simulink model "Older_model_ contains_ACC"  (R2023b)
settings: Solver=VariableStepAuto  StartTime=0.0  StopTime=30  MaxStep=1e-2  RelTol=1e-3  AbsTol=1e-3
values from neighbouring files (symbols this model uses):
  b = 1.6    [a2024_v2x_matlab_6veh.m]
  m = 2000    [a2024_v2x_matlab_6veh.m]
  mEgo = 1500    [a2024_v2x_matlab_6veh.m]
  sampleTime = 0.1    [a2024_v2x_matlab_6veh.m]    (also in v2x_matlab.m; v2x_matlabV2.m; v2x_matlab_6veh.m; v2x_matlab_R.m)
  t_gap = 1.4    [a2024_v2x_matlab_6veh.m]
  waypoints = [egoWP(:,2) egoWP(:,1), zeroforwp]    [a2024_v2x_matlab_6veh.m]    (also in misc.m = data.data.ActorSpecifications(1,1).Waypoints(:,[1,2]); v2x_matlab.m = data.data.ActorSpecifications(1,1).Waypoints(:,[1,2]); v2x_matlabV2.m = [5 -1.6 0; v2x_matlab_R.m = [5 -1.6 0)
  ZeroActors = struct(     'ActorID',0,     'Position', [1000 1000 1000],      'Velocity', [0 0 0],      'Roll', 0,      'Pitch', 0,      'Yaw', 0,      'AngularVelocity', [0 0 0])    [v2x_matlabV2.m]    (also in v2x_matlab_R.m)
undefined symbols (not defined in the file or in its folder): doppler, driving, n, PredictionHorizon, Ts
libraries: simulink x13, simulink_extras x12, commofdm x10, commdigbbndam3 x10, commchan3 x3, drivingscenarioandsensors x3, mpcadaslib x2, commsink2 x2, vehdynlibdriver x1, dspmathops x1, autolibshared x1
(part 2 of 3)

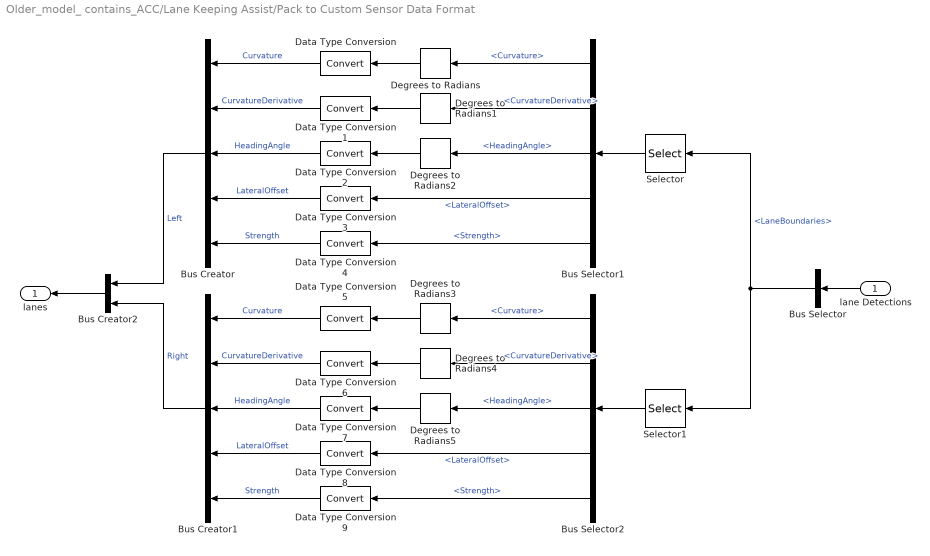
== system Older_model_ contains_ACC/Lane Keeping Assist/Pack to Custom Sensor Data Format ==
  lane Detections : Inport
  Bus Creator : BusCreator  Inputs=5
  Bus Creator1 : BusCreator  Inputs=5
  Bus Creator2 : BusCreator  Inputs=2
  Bus Selector : BusSelector  OutputSignals=LaneBoundaries
  Bus Selector1 : BusSelector  OutputSignals=Curvature,CurvatureDerivative,HeadingAngle,LateralOffset,Strength
  Bus Selector2 : BusSelector  OutputSignals=Curvature,CurvatureDerivative,HeadingAngle,LateralOffset,Strength
  Data Type Conversion{,1..9} (10 alike) : DataTypeConversion  SaturateOnIntegerOverflow=off  RndMeth=Floor
  Degrees to Radians{,1..5} (6 alike) : simulink_extras/Transformations/Degrees to Radians
  Selector : Selector  IndexMode=Zero-based  InputPortWidth=30  IndexOptions=Index vector (dialog)  Indices=1  OutputSizes=1
  Selector1 : Selector  InputPortWidth=30  IndexOptions=Index vector (dialog)  Indices=2  OutputSizes=1
  lanes : Outport  VectorParamsAs1DForOutWhenUnconnected=off
  wires:
  lane Detections/1 -> Bus Selector/1
  Bus Selector/1 -> Selector/1, Selector1/1  "<LaneBoundaries>"
  Selector/1 -> Bus Selector1/1
  Bus Selector1/2 -> Degrees to Radians1/1  "<CurvatureDerivative>"
  Bus Selector1/1 -> Degrees to Radians/1  "<Curvature>"
  Bus Selector1/3 -> Degrees to Radians2/1  "<HeadingAngle>"
  Degrees to Radians/1 -> Data Type Conversion/1
  Degrees to Radians1/1 -> Data Type Conversion1/1
  Degrees to Radians2/1 -> Data Type Conversion2/1
  Bus Selector1/4 -> Data Type Conversion3/1  "<LateralOffset>"
  Bus Selector1/5 -> Data Type Conversion4/1  "<Strength>"
  Data Type Conversion/1 -> Bus Creator/1  "Curvature"
  Data Type Conversion1/1 -> Bus Creator/2  "CurvatureDerivative"
  Data Type Conversion2/1 -> Bus Creator/3  "HeadingAngle"
  Data Type Conversion3/1 -> Bus Creator/4  "LateralOffset"
  Data Type Conversion4/1 -> Bus Creator/5  "Strength"
  Data Type Conversion9/1 -> Bus Creator1/5  "Strength"
  Data Type Conversion6/1 -> Bus Creator1/2  "CurvatureDerivative"
  Data Type Conversion7/1 -> Bus Creator1/3  "HeadingAngle"
  Data Type Conversion8/1 -> Bus Creator1/4  "LateralOffset"
  Data Type Conversion5/1 -> Bus Creator1/1  "Curvature"
  Bus Selector2/1 -> Degrees to Radians3/1  "<Curvature>"
  Selector1/1 -> Bus Selector2/1
  Bus Selector2/4 -> Data Type Conversion8/1  "<LateralOffset>"
  Bus Selector2/5 -> Data Type Conversion9/1  "<Strength>"
  Bus Selector2/2 -> Degrees to Radians4/1  "<CurvatureDerivative>"
  Degrees to Radians5/1 -> Data Type Conversion7/1
  Degrees to Radians3/1 -> Data Type Conversion5/1
  Degrees to Radians4/1 -> Data Type Conversion6/1
  Bus Selector2/3 -> Degrees to Radians5/1  "<HeadingAngle>"
  Bus Creator2/1 -> lanes/1
  Bus Creator/1 -> Bus Creator2/1  "Left"
  Bus Creator1/1 -> Bus Creator2/2  "Right"

== system Older_model_ contains_ACC/Lane Keeping Assist/Subsystem ==
  Lane Assist Offset : Inport
  Lane Sensor data : Inport  Port=2
  Bus Selector3 : BusSelector  OutputSignals=Left.LateralOffset,Right.LateralOffset
  Gain3 : Gain  Gain=-1
  Logical Operator : Logic  Operator=OR  AllPortsSameDT=off  OutDataTypeStr=boolean
  Relational Operator : RelationalOperator  Operator=<=  OutDataTypeStr=boolean  RndMeth=Simplest  InputSameDT=off
  Relational Operator1 : RelationalOperator  OutDataTypeStr=boolean  RndMeth=Simplest  InputSameDT=off
  Departure Detected : Outport
  wires:
  Relational Operator1/1 -> Logical Operator/2
  Bus Selector3/2 -> Relational Operator1/1  "<LateralOffset>"
  Bus Selector3/1 -> Relational Operator/1  "<LateralOffset>"
  Relational Operator/1 -> Logical Operator/1
  Logical Operator/1 -> Departure Detected/1
  Gain3/1 -> Relational Operator1/2
  Lane Assist Offset/1 -> Gain3/1, Relational Operator/2
  Lane Sensor data/1 -> Bus Selector3/1

== system Older_model_ contains_ACC/Lane Keeping Assist/Subsystem2 ==
  Enable : Inport
  Set : Inport  Port=2
  Assisted Steer : Inport  Port=3
  Driver Steer : Inport  Port=4
  AND : Logic  IconShape=distinctive  AllPortsSameDT=off  OutDataTypeStr=boolean
  Latch Assist : Subsystem
  Subsystem1 : Subsystem
  Switch : Switch  Criteria=u2 > Threshold  SaturateOnIntegerOverflow=off  InputSameDT=off
  Status : Outport
  SteeringAngle in rad : Outport  Port=2
  wires:
  Enable/1 -> AND/1
  AND/1 -> Status/1, Switch/2
  Latch Assist/1(Assist) -> AND/2
  Subsystem1/1(Similar) -> Latch Assist/2(Reset)
  Driver Steer/1 -> Switch/3, Subsystem1/2(Driver Steer)
  Assisted Steer/1 -> Switch/1, Subsystem1/1(Assisted Steer)
  Switch/1 -> SteeringAngle in rad/1
  Set/1 -> Latch Assist/1(Set)

== system Older_model_ contains_ACC/Subsystem3/If Action Subsystem ==
  In1 : Inport
  Action Port : ActionPort  ActionPortLabel=case [ 1 ]:
  Out1 : Outport
  wires:
  In1/1 -> Out1/1

== system Older_model_ contains_ACC/Subsystem3/If Action Subsystem1 ==
  In1 : Inport
  Action Port : ActionPort  ActionPortLabel=case [ 2 ]:
  Out1 : Outport
  wires:
  In1/1 -> Out1/1

== system Older_model_ contains_ACC/Subsystem3/If Action Subsystem2 ==
  Actors : Inport
  Action Port : ActionPort  ActionPortLabel=case [ 3 ]:
  Out1 : Outport
  wires:
  Actors/1 -> Out1/1

== system Older_model_ contains_ACC/Subsystem3/If Action Subsystem3 ==
  Actors : Inport
  Action Port : ActionPort  ActionPortLabel=case [ 4 ]:
  Out1 : Outport
  wires:
  Actors/1 -> Out1/1

== system Older_model_ contains_ACC/Subsystem3/If Action Subsystem4 ==
  Actors : Inport
  Action Port : ActionPort  ActionPortLabel=case [ 5 ]:
  Out1 : Outport
  wires:
  Actors/1 -> Out1/1

== system Older_model_ contains_ACC/Subsystem3/Subsystem1 ==
  In1 : Inport
  Bit to Integer Converter2 : simulink/Logic and Bit Operations/Bit to Integer Converter  nbits=16  bitOrder=MSB first  signedOutputValues=Signed  outDtype=int16  outDtypeSigned=int16
  MATLAB Function3 : MATLAB Function  TreatAsAtomicUnit=on
  OFDM Demodulator : commofdm/OFDM Demodulator  StatePerturbationForJacobian=1.0e-05  FFTLength=64  NumGuardBandCarriers=[0; 0]  RemoveDCCarrier=on  PilotOutputPort=on  PilotCarrierIndices=[12; 26; 40; 54]  CyclicPrefixLength=32  OversamplingFactor=3  NumSymbols=1  NumReceiveAntennas=1  SimulateUsing=Interpreted execution
  Rectangular QAM Demodulator Baseband2 : commdigbbndam3/Rectangular QAM Demodulator Baseband  M=2^6  OutType=Bit  DecType=Hard decision  VarSource=Dialog  Variance=1  Dec=Binary  Mapping=[0:15]  PowType=Average Power  MinDist=2  AvgPow=P_Signal  PeakPow=1  Ph=0  outDtype1=int16  outDtype2=int16  derotateFactorWordLen=16  derotateFactorDataTypeStr=Inherit: Same word length as input  derotateFactorLastDataTypeStr=Inherit: Same word length as input  denormFactorWordLen=16  denormFactorDataTypeStr=Inherit: Same word length as input  denormFactorLastDataTypeStr=Inherit: Same word length as input  prodOutWordLen=32  prodOutOverflowMode=Wrap  prodOutRoundingMode=Floor  prodOutOvFlMode=off  prodOutOvFlModeLastStrValue=off  sumWordLen=32
      settings: LibrarySourceBlock=|
      | commhdldigbbndam/Rectangular QAM
      | Demodulator
      | Baseband
  Terminator : Terminator
  To Workspace : ToWorkspace  VariableName=demodulated  SampleTime=-1
  input : Outport
  wires:
  In1/1 -> OFDM Demodulator/1
  Rectangular QAM Demodulator Baseband2/1 -> Bit to Integer Converter2/1
  MATLAB Function3/1(output) -> Rectangular QAM Demodulator Baseband2/1
  OFDM Demodulator/1 -> MATLAB Function3/1(input)  "Before QAM Demod"
  Bit to Integer Converter2/1 -> To Workspace/1, input/1
  OFDM Demodulator/2 -> Terminator/1

== system Older_model_ contains_ACC/Lane Keeping Assist/Estimate lane center/Center from None ==
  lanes : Inport
  Trigger : TriggerPort  TriggerType=function-call  VariantControl=(inherit)  PortDimensions=1
  Out1 : Outport
  wires:
  lanes/1 -> Out1/1

== system Older_model_ contains_ACC/Lane Keeping Assist/Estimate lane center/Center from left ==
  note: Curvature
      | = 1 / ( 1 / (left curvature) – guard)
      | = left curvature / (1 – (left curvature) * guard).
  note: Curvature Derivative
      | = D[ 1 / ( 1 / (left curvature) – guard)]
      | = left curvature derivative / (1 – (left curvature) * guard)^2.
  Lanes : Inport
  Trigger : TriggerPort  TriggerType=function-call  VariantControl=(inherit)  PortDimensions=1
  Add : Sum  Inputs=+-
  Add1 : Sum  Inputs=+-
  Bus Creator1 : BusCreator  Inputs=4  OutDataTypeStr=Bus: InternalBuses
      settings: InheritFromInputs=off
  Bus Selector3 : BusSelector  OutputSignals=Left.Curvature,Left.CurvatureDerivative,Left.HeadingAngle,Left.LateralOffset
  Constant4 : Constant  Value=2
  Constant7 : Constant
  Constant8 : Constant  Value=2
  Divide : Product  Inputs=*/
  Divide1 : Product  Inputs=*/
  Product : Product
  Square : Math  Operator=square
  Center : Outport
  wires:
  Bus Selector3/4 -> Add1/1  "<LateralOffset>"
  Bus Selector3/1 -> Divide/1, Product/1  "<Curvature>"
  Add1/1 -> Bus Creator1/4
  Divide/1 -> Bus Creator1/1
  Constant7/1 -> Add/1
  Constant4/1 -> Product/2
  Add/1 -> Divide/2, Square/1
  Product/1 -> Add/2
  Divide1/1 -> Bus Creator1/2
  Lanes/1 -> Bus Selector3/1
  Bus Selector3/2 -> Divide1/1  "<CurvatureDerivative>"
  Bus Selector3/3 -> Bus Creator1/3  "<HeadingAngle>"
  Constant8/1 -> Add1/2
  Square/1 -> Divide1/2
  Bus Creator1/1 -> Center/1

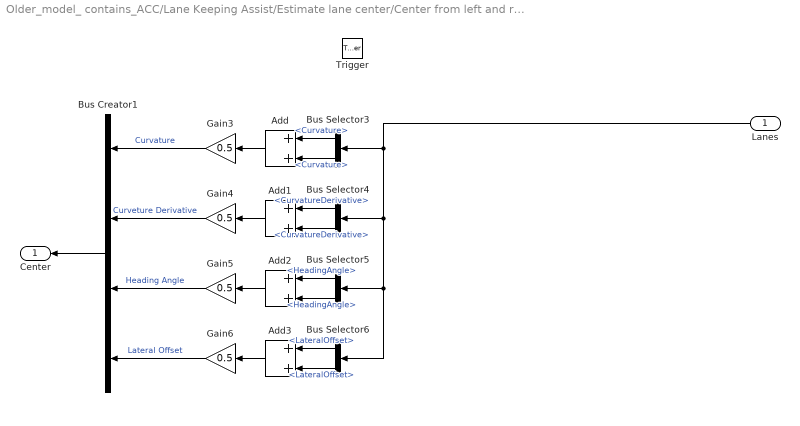
== system Older_model_ contains_ACC/Lane Keeping Assist/Estimate lane center/Center from left and right ==
  Lanes : Inport
  Trigger : TriggerPort  TriggerType=function-call  VariantControl=(inherit)  PortDimensions=1
  Add{,1..3} (4 alike) : Sum
  Bus Creator1 : BusCreator  Inputs=4  OutDataTypeStr=Bus: InternalBuses
      settings: InheritFromInputs=off
  Bus Selector3 : BusSelector  OutputSignals=Left.Curvature,Right.Curvature
  Bus Selector4 : BusSelector  OutputSignals=Left.CurvatureDerivative,Right.CurvatureDerivative
  Bus Selector5 : BusSelector  OutputSignals=Left.HeadingAngle,Right.HeadingAngle
  Bus Selector6 : BusSelector  OutputSignals=Left.LateralOffset,Right.LateralOffset
  Gain{3..6} (4 alike) : Gain  Gain=0.5
  Center : Outport
  wires:
  Add1/1 -> Gain4/1
  Bus Selector3/1 -> Add/1  "<Curvature>"
  Gain4/1 -> Bus Creator1/2  "Curveture Derivative"
  Bus Selector5/1 -> Add2/1  "<HeadingAngle>"
  Gain3/1 -> Bus Creator1/1  "Curvature"
  Lanes/1 -> Bus Selector6/1, Bus Selector5/1, Bus Selector4/1, Bus Selector3/1
  Bus Selector5/2 -> Add2/2  "<HeadingAngle>"
  Add2/1 -> Gain5/1
  Bus Selector3/2 -> Add/2  "<Curvature>"
  Add/1 -> Gain3/1
  Bus Selector4/1 -> Add1/1  "<CurvatureDerivative>"
  Gain6/1 -> Bus Creator1/4  "Lateral Offset"
  Bus Selector4/2 -> Add1/2  "<CurvatureDerivative>"
  Bus Selector6/2 -> Add3/2  "<LateralOffset>"
  Bus Selector6/1 -> Add3/1  "<LateralOffset>"
  Add3/1 -> Gain6/1
  Gain5/1 -> Bus Creator1/3  "Heading Angle"
  Bus Creator1/1 -> Center/1

== system Older_model_ contains_ACC/Lane Keeping Assist/Estimate lane center/Center from right ==
  note: Curvature
      | = 1 / ( 1 / (right curvature) – guard)
      | = right curvature / (1 – (right curvature) * guard).
  note: Curvature Derivative
      | = D[ 1 / ( 1 / (right curvature) – guard)]
      | = right curvature derivative / (1 – (right curvature) * guard)^2.
  Lanes : Inport
  Trigger : TriggerPort  TriggerType=function-call  VariantControl=(inherit)  PortDimensions=1
  Add : Sum  Inputs=+-
  Add1 : Sum  Inputs=+-
  Bus Creator1 : BusCreator  Inputs=4  OutDataTypeStr=Bus: InternalBuses
      settings: InheritFromInputs=off
  Bus Selector3 : BusSelector  OutputSignals=Right.Curvature,Right.CurvatureDerivative,Right.HeadingAngle,Right.LateralOffset
  Constant4 : Constant  Value=2
  Constant7 : Constant
  Constant8 : Constant  Value=2
  Divide : Product  Inputs=*/
  Divide1 : Product  Inputs=*/
  Product : Product
  Square : Math  Operator=square
  Center : Outport
  wires:
  Bus Selector3/4 -> Add1/1  "<LateralOffset>"
  Bus Selector3/1 -> Divide/1, Product/1  "<Curvature>"
  Add1/1 -> Bus Creator1/4
  Divide/1 -> Bus Creator1/1
  Constant7/1 -> Add/1
  Constant4/1 -> Product/2
  Add/1 -> Divide/2, Square/1
  Product/1 -> Add/2
  Divide1/1 -> Bus Creator1/2
  Lanes/1 -> Bus Selector3/1
  Bus Selector3/2 -> Divide1/1  "<CurvatureDerivative>"
  Bus Selector3/3 -> Bus Creator1/3  "<HeadingAngle>"
  Constant8/1 -> Add1/2
  Square/1 -> Divide1/2
  Bus Creator1/1 -> Center/1

== system Older_model_ contains_ACC/Lane Keeping Assist/Subsystem2/Latch Assist ==
  Set : Inport
  Reset : Inport  Port=2
  AND : Logic  IconShape=distinctive  AllPortsSameDT=off  OutDataTypeStr=boolean
  Delay : Delay  DelayLength=1
  NOT : Logic  Operator=NOT  IconShape=distinctive  AllPortsSameDT=off  OutDataTypeStr=boolean
  OR : Logic  Operator=OR  IconShape=distinctive  AllPortsSameDT=off  OutDataTypeStr=boolean
  Assist : Outport  VectorParamsAs1DForOutWhenUnconnected=off
  wires:
  Reset/1 -> NOT/1
  NOT/1 -> AND/1
  Set/1 -> OR/1
  OR/1 -> Delay/1, Assist/1
  Delay/1 -> AND/2
  AND/1 -> OR/2

== system Older_model_ contains_ACC/Lane Keeping Assist/Subsystem2/Subsystem1 ==
  Assisted Steer : Inport
  Driver Steer : Inport  Port=2
  Abs : Abs  SaturateOnIntegerOverflow=off
  Add : Sum  Inputs=+-
  Constant3 : Constant  Value=0.1
  Data Type Conversion : DataTypeConversion  OutDataTypeStr=single  SaturateOnIntegerOverflow=off  RndMeth=Floor
  Deteted 5 Similar Steer Values : simulink/Logic and Bit Operations/Compare To Constant  relop=>=  const=5  OutDataTypeStr=boolean
  Relational Operator : RelationalOperator  Operator=<=  OutDataTypeStr=boolean  RndMeth=Simplest  InputSameDT=off
  Sum of Elements : Sum  Inputs=+
  Tapped Delay : simulink/Discrete/Tapped Delay  vinit=0.0  samptime=-1  NumDelays=5  DelayOrder=Oldest  includeCurrent=off
  Similar : Outport
  wires:
  Relational Operator/1 -> Data Type Conversion/1
  Abs/1 -> Relational Operator/1
  Add/1 -> Abs/1
  Tapped Delay/1 -> Sum of Elements/1
  Constant3/1 -> Relational Operator/2
  Data Type Conversion/1 -> Tapped Delay/1
  Driver Steer/1 -> Add/2
  Assisted Steer/1 -> Add/1
  Sum of Elements/1 -> Deteted 5 Similar Steer Values/1
  Deteted 5 Similar Steer Values/1 -> Similar/1

== matlab function Older_model_ contains_ACC/MATLAB Function2 ==
  settings: sampleTime=sampleTime
  data: u input; y output double
function y = fcn(u)

if isempty(u) 
    y = zeros(1,15);
else
    y = double(u);
end

end

== matlab function Older_model_ contains_ACC/Subsystem/MATLAB Function ==
  settings: updateMethod=DISCRETE  sampleTime=sampleTime
  data: modulated input; signal output; SNR input
function signal = PRO_error(modulated, SNR)

signal = awgn(modulated,SNR);

== matlab function Older_model_ contains_ACC/Subsystem5/MATLAB Function ==
  data: modulated input; signal output; SNR input
function signal = PRO_error(modulated, SNR)

signal = awgn(modulated,SNR);

end

== matlab function Older_model_ contains_ACC/Subsystem5/MATLAB Function1 ==
  data: busActors3Test1 input; Actor output int16 size=15; VehicleID input; VehicleData output Bus: Actors; EgoData input Bus: Actors; counter output; SNR output
  events: trigger input RISING_EDGE_EVENT
function [Actor, VehicleData, counter, SNR]  = convBus2IntVector(busActors3Test1, VehicleID, EgoData)

% Data extracted from actorss bus

%ActorId = BusActors1Actors.Actors(ActorID).ActorID(1:1);
numActors = busActors3Test1.NumActors;
%time = busActors3Test1.Time;
time = busActors3Test1.Time;

ActorID = VehicleID;

posX = busActors3Test1.Actors(ActorID).Position(1:1);
posY = busActors3Test1.Actors(ActorID).Position(2:2);
posZ = busActors3Test1.Actors(ActorID).Position(3:3);
vPos = [posX posY posZ];

vX = busActors3Test1.Actors(ActorID).Velocity(1:1);
vY = busActors3Test1.Actors(ActorID).Velocity(2:2);
vZ = busActors3Test1.Actors(ActorID).Velocity(3:3);

roll = busActors3Test1.Actors(ActorID).Roll(1:1);
pitch = busActors3Test1.Actors(ActorID).Pitch(1:1);
yaw = busActors3Test1.Actors(ActorID).Yaw(1:1);


angularVelocityX = busActors3Test1.Actors(ActorID).AngularVelocity(1:1);
angularVelocityY = busActors3Test1.Actors(ActorID).AngularVelocity(2:2);
angularVelocityZ = busActors3Test1.Actors(ActorID).AngularVelocity(3:3);

VehicleData = busActors3Test1.Actors(ActorID);


%% Converting the data

ActorID = int16(ActorID);

posMultip = 10;
posX = int16(round(posMultip*posX));
posY = int16(round(posMultip*posY));
posZ = int16(round(posMultip*posZ));

velMultip = 50;
vX = int16(round(velMultip * vX));
vY = int16(round(velMultip * vY));
vZ = int16(round(velMultip * vZ));

rpyMultip = 50;
roll = int16(round(rpyMultip * roll));
pitch = int16(round(rpyMultip * pitch));
yaw = int16(round(rpyMultip * yaw));

angvelMultip = 50;
angularVelocityX = int16(round(angvelMultip * angularVelocityX));
angularVelocityY = int16(round(angvelMultip * angularVelocityY));
angularVelocityZ = int16(round(angvelMultip * angularVelocityZ));


% Output vector
%zerosVector = zeros(9,1);

intVector = [numActors; time; ActorID; posX; posY; posZ; vX; vY; vZ; roll; pitch; yaw; angularVelocityX; angularVelocityY; angularVelocityZ];



%% Pathloss (freespace)

EgoPos = EgoData.Position;
dist = abs(norm(vPos) - norm(EgoPos));

fc = 5.9*10^9;  % Carrier frequency
lambda = physconst('LightSpeed')/fc;

PL = fspl(dist, lambda);



Pt_dBm = 33;    % [dBm] Transmission power; maximum permissible transmit power level
sigma = rand(1) + 3.2;  % [3.7 +- 0.5] Variance of the shadowing effect in the wireless communication channel
                        % shadowing follows a log-normal random distribution
X = 2*rand(1)-1;     % random variable following a normal distribution with mean 0 and standard deviation 1
SH = sigma * X;

Pr = Pt_dBm - PL - SH;

P_SEN = -50;

%ZeroActors = int16(zeros(15,1));


counter = 0;
% storedPacket = int16(nan(15,1));
% 
% if Pr > P_SEN
%     Actor = intVector;
%     storedPacket = intVector;
%     counter = 0;
% elseif counter < 10
%     Actor = storedPacket;
%     counter = counter + 1;
% else (counter > 10 & counter == 10)
%     Actor = int16(nan(15,1));
% end

%disp(storedPacket)


persistent prev_value;
if isempty(prev_value)
    prev_value = int16(nan(15,1)); % Initialize to a default value
end

if Pr > P_SEN
    Actor = intVector;
    prev_value = intVector;
    counter = 0;
elseif counter < 1
    Actor = prev_value;
    counter = counter + 1;
end

%% SNR

F = 6; % [dB] Noise figure
k = physconst('Boltzmann'); % Boltzmann állandó
T = 300; % [K] Abszolút hőmérséklet

N0 = F*k*T;

SNR = Pt_dBm - N0;


%% Packet counter
counter = 0;

if (Pr > P_SEN)
    counter = counter + 1;
end


end

== matlab function Older_model_ contains_ACC/Channel/MATLAB Function1 ==
  data: Actors output Bus: Actors; ActorsIn input; Positions output; Distances output; Ego input
function [Actors, Positions, Distances] = SelectActor(ActorsIn, Ego)

EgoActor = Ego;
Actors = ActorsIn.Actors;


% Separating
Lead = ActorsIn.Actors(1);
Interfering = ActorsIn.Actors(3);
Threshold = ActorsIn.Actors(2);

% Distances
EgoPos = Ego.Position';
LeadPos = Lead.Position';
InterferingPos = Interfering.Position';
ThresholdPos = Threshold.Position';

Positions = [EgoPos LeadPos InterferingPos ThresholdPos];

%EgoDists
EgoDist = [norm(EgoPos-EgoPos);
            norm(EgoPos-LeadPos);
            norm(EgoPos-InterferingPos);
            norm(EgoPos-ThresholdPos)];

%LeadDists
LeadDist = [norm(LeadPos-EgoPos);
            norm(LeadPos-LeadPos);
            norm(LeadPos-InterferingPos);
            norm(LeadPos-ThresholdPos)];

%InterferringDists
InterferringDist = [norm(InterferingPos-EgoPos);
                    norm(InterferingPos-LeadPos);
                    norm(InterferingPos-InterferingPos);
                    norm(InterferingPos-ThresholdPos)];

% ThresholdDists
ThresholdDist = [norm(ThresholdPos-EgoPos);
                norm(ThresholdPos-LeadPos);
                norm(ThresholdPos-InterferingPos);
                norm(ThresholdPos-ThresholdPos)];


Distances = [EgoDist, LeadDist, InterferringDist, ThresholdDist] ;

end

== matlab function Older_model_ contains_ACC/Subsystem4/MATLAB Function ==
  data: modulated input; signal output; SNR input
function signal = PRO_error(modulated, SNR)

signal = awgn(modulated,SNR);

== matlab function Older_model_ contains_ACC/Subsystem4/MATLAB Function1 ==
  data: busActors3Test1 input; Actor output int16 size=15; VehicleID input; VehicleData output Bus: Actors; EgoData input Bus: Actors; counter output; SNR output
  events: trigger input RISING_EDGE_EVENT
function [Actor, VehicleData, counter, SNR]  = convBus2IntVector(busActors3Test1, VehicleID, EgoData)

% Data extracted from actorss bus

%ActorId = BusActors1Actors.Actors(ActorID).ActorID(1:1);
numActors = busActors3Test1.NumActors;
%time = busActors3Test1.Time;
time = busActors3Test1.Time;

ActorID = VehicleID;

posX = busActors3Test1.Actors(ActorID).Position(1:1);
posY = busActors3Test1.Actors(ActorID).Position(2:2);
posZ = busActors3Test1.Actors(ActorID).Position(3:3);
vPos = [posX posY posZ];

vX = busActors3Test1.Actors(ActorID).Velocity(1:1);
vY = busActors3Test1.Actors(ActorID).Velocity(2:2);
vZ = busActors3Test1.Actors(ActorID).Velocity(3:3);

roll = busActors3Test1.Actors(ActorID).Roll(1:1);
pitch = busActors3Test1.Actors(ActorID).Pitch(1:1);
yaw = busActors3Test1.Actors(ActorID).Yaw(1:1);


angularVelocityX = busActors3Test1.Actors(ActorID).AngularVelocity(1:1);
angularVelocityY = busActors3Test1.Actors(ActorID).AngularVelocity(2:2);
angularVelocityZ = busActors3Test1.Actors(ActorID).AngularVelocity(3:3);

VehicleData = busActors3Test1.Actors(ActorID);


%% Converting the data

ActorID = int16(ActorID);

posMultip = 10;
posX = int16(round(posMultip*posX));
posY = int16(round(posMultip*posY));
posZ = int16(round(posMultip*posZ));

velMultip = 50;
vX = int16(round(velMultip * vX));
vY = int16(round(velMultip * vY));
vZ = int16(round(velMultip * vZ));

rpyMultip = 50;
roll = int16(round(rpyMultip * roll));
pitch = int16(round(rpyMultip * pitch));
yaw = int16(round(rpyMultip * yaw));

angvelMultip = 50;
angularVelocityX = int16(round(angvelMultip * angularVelocityX));
angularVelocityY = int16(round(angvelMultip * angularVelocityY));
angularVelocityZ = int16(round(angvelMultip * angularVelocityZ));


% Output vector
%zerosVector = zeros(9,1);

intVector = [numActors; time; ActorID; posX; posY; posZ; vX; vY; vZ; roll; pitch; yaw; angularVelocityX; angularVelocityY; angularVelocityZ];



%% Pathloss (freespace)

EgoPos = EgoData.Position;
dist = norm(vPos - EgoPos);

fc = 5.9*10^9;  % Carrier frequency
lambda = physconst('LightSpeed')/fc;

PL = fspl(dist, lambda);

Pt_dBm = 33;    % [dBm] Transmission power; maximum permissible transmit power level
sigma = rand(1) + 3.2;  % [3.7 +- 0.5] Variance of the shadowing effect in the wireless communication channel
                        % shadowing follows a log-normal random distribution
X = 2*rand(1)-1;       % random variable following a normal distribution with mean 0 and standard deviation 1
SH = sigma * X;

Pr = Pt_dBm - PL - SH;

P_SEN = -60;

%ZeroActors = int16(zeros(15,1));

counter = 0;
% storedPacket = int16(nan(15,1));
% 
% if Pr > P_SEN
%     Actor = intVector;
%     storedPacket = intVector;
%     counter = 0;
% elseif counter < 10
%     Actor = storedPacket;
%     counter = counter + 1;
% else 
%     Actor = int16(nan(15,1));
% end
%disp(storedPacket)


persistent prev_value;
if isempty(prev_value)
    prev_value = int16(nan(15,1)); % Initialize to a default value
end

if Pr > P_SEN
    Actor = intVector;
    prev_value = intVector;
    counter = 0;
elseif counter < 1
    Actor = prev_value;
    counter = counter + 1;
end

%% SNR

F = 6; % [dB] Noise figure
k = physconst('Boltzmann'); % Boltzmann 
T = 300; % [K] Absolut temperature

N0 = F*k*T;

SNR = Pt_dBm - N0;


%% Packet counter
counter = 0;

if (Pr > P_SEN)
    counter = counter + 1;
end


end

== matlab function Older_model_ contains_ACC/Channel/MATLAB Function9 ==
  data: Ego input; Actors input Bus: Actors; LeadActor output Bus: Actors size=1; InterferingActor output Bus: Actors size=1; ThresholdActor output Bus: Actors size=1; PSR output; Positions input; ZeroActors input
function [LeadActor,InterferingActor,ThresholdActor,PSR] = SEN_PSR(Ego, Actors, Positions, ZeroActors)
coder.extrinsic('Simulink.Bus')

%% Extract data
Lead = Actors(1);
Interfering = Actors(2);
Threshold = Actors(3);

EgoPos = Positions(:,1);
LeadPos = Positions(:,2);
InterferingPos = Positions(:,3);
ThresholdPos = Positions(:,4);

%% Calculating distances
de_lead = norm(LeadPos - EgoPos);                % Ego-Lead Distance
de_interfering = norm(InterferingPos - EgoPos);  % Ego-Interferring Distance
de_threshold = norm(ThresholdPos  - EgoPos);     % Ego-Threshold distance

dl_interfering = norm(InterferingPos - LeadPos);
dl_threshold = norm(ThresholdPos - LeadPos);

di_threshold = norm(ThresholdPos - InterferingPos);

%% Pathloss (freespace)
fc = 5.9*10^9;  % Carrier frequency
lambda = physconst('LightSpeed')/fc;

PL_EL = fspl(de_lead, lambda);
PL_EI = fspl(de_interfering, lambda);
PL_ET = fspl(de_threshold, lambda);

PL_LI = fspl(dl_interfering, lambda);
PL_LT = fspl(dl_threshold, lambda);

PL_IT = fspl(di_threshold, lambda);


% Transmission Power (Pt)
Pt_dBm = 33;    % [dBm] Transmission power; maximum permissible transmit power level
%Pt_dBw = Pt_dBm - 30; % [dBw]
%Pt_watts = (10 .^ (dBm / 10))/1000;  % Transmission power in W

sigma = rand(1) + 3.2;  % [3.7 +- 0.5] Variance of the shadowing effect in the wireless communication channel
                        % shadowing follows a log-normal random distribution
X = randn(1);       % random variable following a normal distribution with mean 0 and standard deviation 1
SH = sigma * X;
Pr_EL = Pt_dBm - PL_EL - SH; 
Pr_EI = Pt_dBm - PL_EI - SH;
Pr_ET = Pt_dBm - PL_ET - SH;

Pr_LI = Pt_dBm - PL_LI  - SH;
Pr_LT = Pt_dBm - PL_LT  - SH;

Pr_IT = Pt_dBm - PL_IT  - SH;


P_SEN = -60;  % [dBm] Sensing threshold
% P_SEN_dBW = P_SEN + 30;

% Lead
persistent prev_value_lead;
if isempty(prev_value_lead)
    prev_value_lead = ZeroActors; % Initialize to a default value
end

if Pr_EL > P_SEN
    LeadActor = Lead;
    prev_value_lead = Lead;
else
    LeadActor = prev_value_lead;
end

% Interfering
%InterferingActorOut = struct;

persistent prev_value_int;
if isempty(prev_value_int)
    prev_value_int = ZeroActors; % Initialize to a default value
end

if Pr_EI > P_SEN
    InterferingActor = Interfering;
    prev_value_int = Interfering;
else
    InterferingActor = prev_value_int;
end

% Threshold
persistent prev_value_thr;


if isempty(prev_value_thr)
    prev_value_thr = ZeroActors; % Initialize to a default value
end

if Pr_ET > P_SEN
    ThresholdActor = Threshold;
    prev_value_thr = Threshold;
else
    ThresholdActor = prev_value_thr;
end


%% PSR 
sigmasqrt2 = sigma * sqrt(2);

% Ego - Lead
deltaPtSEN_EL = Pt_dBm - PL_EL - P_SEN;
delta_SEN_EL = 0.5*(1-erf(deltaPtSEN_EL/sigmasqrt2));
PSR_EL = 1-delta_SEN_EL;

% Ego - Interfering
deltaPtSEN_EI = Pt_dBm - PL_EI - P_SEN;
delta_SEN_EI = 0.5*(1-erf(deltaPtSEN_EI/sigmasqrt2));
PSR_EI = 1-delta_SEN_EI;

% Ego - Threshold
deltaPtSEN_ET = Pt_dBm - PL_ET - P_SEN;
delta_SEN_ET = 0.5*(1-erf(deltaPtSEN_ET/sigmasqrt2));
PSR_ET = 1-delta_SEN_ET;

% Lead - Interfering
deltaPtSEN_LI = Pt_dBm - PL_LI - P_SEN;
delta_SEN_LI = 0.5*(1-erf(deltaPtSEN_LI/sigmasqrt2));
PSR_LI = 1-delta_SEN_LI;

% Lead - Threshold
deltaPtSEN_LT = Pt_dBm - PL_LT - P_SEN;
delta_SEN_LT = 0.5*(1-erf(deltaPtSEN_LT/sigmasqrt2));
PSR_LT = 1-delta_SEN_LT;

% Interfering - Threshold;
deltaPtSEN_IT = Pt_dBm - PL_IT - P_SEN;
delta_SEN_IT = 0.5*(1-erf(deltaPtSEN_IT/sigmasqrt2));
PSR_IT = 1-delta_SEN_IT;


PSR = [PSR_EL PSR_EI PSR_ET PSR_LI PSR_LT PSR_IT];

end

== matlab function Older_model_ contains_ACC/Channel/MATLAB Function4 ==
  data: PSR input; CBR output
function CBR = CBR(PSR)

lambda = (1/0.01)*3;            % Packets/second
T = 0.008;                      % Packet duration


beta = 4*4.7/400;   % Traffic density (vehicle/meter)

load_ir = lambda * T * PSR;

% CBR upper bound:
CBR_u = beta * sum(load_ir);    % distance between vehicle vi and the ego vehicle
                                % upper bound, because it does not take into account packet collisions
p1 = -0.2481;
p2 = 0.913;
p3 = 0.003844;

CBR = p1*CBR_u^2 + p2*CBR_u + p3

end

== matlab function Older_model_ contains_ACC/Ego trajectory ==
  settings: updateMethod=DISCRETE  sampleTime=sampleTime
  data: EgoFdbX input; EgoFdbY input; LongRef output; LatRef output; YawRef output; waypoints input
function [LongRef, LatRef, YawRef] = generateTrajectory(EgoFdbX, EgoFdbY, waypoints)

LongFdb = EgoFdbX;
LatFdb = EgoFdbY;
EgoFdb= [LongFdb, LatFdb]; % Ego feedback positions norm

% waypoints = [-104.6000, 6.6000, deg2rad(2.9993);
%             54.7000, -14.8000, deg2rad(-29.0375);
%             91.4000, -42.6000, deg2rad(-44.2776);
%             163.6000, -148.6000, deg2rad(-61.4646)];





count = 1;

min_distance = inf;

for i = 1:size(waypoints, 1)
    RefPose = waypoints(i,1:2);
    distance = norm(RefPose - EgoFdb);

    if abs(distance) < min_distance
        min_distance = abs(distance);
        count = i;
    end
end


if count > size(waypoints, 1)
    count = size(waypoints, 1);  % Ensure count doesn't exceed the number of rows in waypoints
end


LongRef = waypoints(count,1);
LatRef = waypoints(count,2);
YawRef = waypoints(count,3);
Output = [LongRef, LatRef, YawRef];
end


% while count <= size(waypoints, 1)
%     RefPosenorm = norm(waypoints(count,1:2));
%     if EgoFdbnorm < RefPosenorm
%         break;
%     else
%         count = count + 1;
%     end
% end
% 
% if count > size(waypoints, 1)
%     count = size(waypoints, 1);  
% end
% 
% RefPose = waypoints(count,:);
% end

% if 0 <= timevector < 1
%     RefPose = waypoints(1,:);
% elseif 1 <= timevector < 2
%     RefPose = waypoints(2,:);
% elseif 2 <= timevector < 3
%     RefPose = waypoints(3,:);
% elseif 3 <= timevector < 4
%     RefPose = waypoints(4,:);
% elseif 4 <= timevector < 5
%     RefPose = waypoints(5,:);
% elseif 5 <= timevector < 6
%     RefPose = waypoints(6,:);
% elseif 6 <= timevector < 7
%     RefPose = waypoints(7,:);
% elseif 7 <= timevector < 8
%     RefPose = waypoints(8,:);
% elseif 8 <= timevector < 9
%     RefPose = waypoints(9,:);
% elseif 9 <= timevector < 10
%     RefPose = waypoints(10,:);
% elseif 10 <= timevector < 11
%     RefPose = waypoints(11,:);
% end
% 
% end

== matlab function Older_model_ contains_ACC/Lane Keeping Assist/Estimate lane center/MATLAB Function1 ==
  data: Left input Bus: Left; Right input Bus: Right
  events: fcnLeftAndRight output FUNCTION_CALL_EVENT; fcnLeftOnly output FUNCTION_CALL_EVENT; fcnRightOnly output FUNCTION_CALL_EVENT; fcnNone output FUNCTION_CALL_EVENT
function fcn(Left, Right)

leftStrength  = Left.Strength;
rightStrength = Right.Strength;

if (leftStrength > 0) && (rightStrength > 0)
   fcnLeftAndRight();
   
elseif leftStrength > 0
    fcnLeftOnly();
    
elseif rightStrength > 0
    fcnRightOnly();
    
else
    fcnNone();
end

== matlab function Older_model_ contains_ACC/Lane Keeping Assist/Estimate lane center/Preview Curvature ==
  data: rho output; Curvature0 input; dCurvature input; Vx input; sampleTime parameter; PredictionHorizon parameter
function rho = predictCurvature(Curvature0,dCurvature,Vx, sampleTime, PredictionHorizon)
% Curvature0 = initial curvature per unit length                  [1/m]
% dCurvature = (constant) derivative of curvature per unit length [1/m^2]
% CurvatureLength = length for which the clothoid model is valid [m]
% Vx = speed of vehicle

% We want to export a set of curvatures at a uniform sample time ahead.
% t is this vector which goes up to 1 second in the future or having
% enough time to reach the known length in curvature (whichever is smaller)

% To enable truncation by curvelength, mark output "rho" as varsize
%t = 0:Ts:min(1,CurvatureLength/Vx);

t = zeros(PredictionHorizon+1,1);
for i=1:numel(t)
    t(i) = (i-1).*sampleTime;
end

% We compute the curvature vector rho(t) using the specified clothoid model
rho = Curvature0 + dCurvature*Vx*t;

== matlab function Older_model_ contains_ACC/Vehicle 2/MATLAB Function1 ==
  data: busActors3Test1 input; intVector output int16 size=15; VehicleID input
  events: trigger input RISING_EDGE_EVENT
function intVector = convBus2IntVector(busActors3Test1, VehicleID)

% Data extracted from actorss bus

%ActorId = BusActors1Actors.Actors(ActorID).ActorID(1:1);
numActors = busActors3Test1.NumActors;
time = busActors3Test1.Time;

ActorID = VehicleID;

posX = busActors3Test1.Actors(ActorID).Position(1:1);
posY = busActors3Test1.Actors(ActorID).Position(2:2);
posZ = busActors3Test1.Actors(ActorID).Position(3:3);

vX = busActors3Test1.Actors(ActorID).Velocity(1:1);
vY = busActors3Test1.Actors(ActorID).Velocity(2:2);
vZ = busActors3Test1.Actors(ActorID).Velocity(3:3);

roll = busActors3Test1.Actors(ActorID).Roll(1:1);
pitch = busActors3Test1.Actors(ActorID).Pitch(1:1);
yaw = busActors3Test1.Actors(ActorID).Yaw(1:1);


angularVelocityX = busActors3Test1.Actors(ActorID).AngularVelocity(1:1);
angularVelocityY = busActors3Test1.Actors(ActorID).AngularVelocity(2:2);
angularVelocityZ = busActors3Test1.Actors(ActorID).AngularVelocity(3:3);


% Converting the data

ActorID = int16(ActorID);

posMultip = 10;
posX = int16(round(posMultip*posX));
posY = int16(round(posMultip*posY));
posZ = int16(round(posMultip*posZ));

velMultip = 50;
vX = int16(round(velMultip * vX));
vY = int16(round(velMultip * vY));
vZ = int16(round(velMultip * vZ));

rpyMultip = 50;
roll = int16(round(rpyMultip * roll));
pitch = int16(round(rpyMultip * pitch));
yaw = int16(round(rpyMultip * yaw));

angvelMultip = 50;
angularVelocityX = int16(round(angvelMultip * angularVelocityX));
angularVelocityY = int16(round(angvelMultip * angularVelocityY));
angularVelocityZ = int16(round(angvelMultip * angularVelocityZ));


% Output vector
%zerosVector = zeros(9,1);

intVector = [numActors; time; ActorID; posX; posY; posZ; vX; vY; vZ; roll; pitch; yaw; angularVelocityX; angularVelocityY; angularVelocityZ];
end

== matlab function Older_model_ contains_ACC/MATLAB Function1 ==
  settings: updateMethod=DISCRETE  sampleTime=sampleTime
  data: xdotin input; y output
function y = initialVelocity(xdotin)

if isempty(xdotin) == true
    y = 16;
elseif xdotin == 0
    y = 16;
else
    y = abs(xdotin);
end

end

== matlab function Older_model_ contains_ACC/MATLAB Function3 ==
  settings: updateMethod=DISCRETE  sampleTime=sampleTime
  data: EgoActor input; busActors3Test1 input; Dist output
function Dist = fcn(EgoActor, busActors3Test1)

EgoPos = EgoActor.Position;

Position1  = double(busActors3Test1.Actors(1).Position);
Position2  = double(busActors3Test1.Actors(2).Position);
Position3  = double(busActors3Test1.Actors(3).Position);
Position4  = double(busActors3Test1.Actors(4).Position);
Position5  = double(busActors3Test1.Actors(5).Position);

Dist1 = norm(EgoPos-Position1);
Dist2 = norm(EgoPos-Position2);
Dist3 = norm(EgoPos-Position3);
Dist4 = norm(EgoPos-Position4);
Dist5 = norm(EgoPos-Position5);

Dist = [Dist1; Dist2; Dist3; Dist4; Dist5]

end

== matlab function Older_model_ contains_ACC/MATLAB Function4 ==
  settings: updateMethod=DISCRETE  sampleTime=sampleTime
  data: u input; RelVel output
function RelVel = fcn(u)

for i = 1:5
    RelVel = 0;
end

RelVel = u;

== matlab function Older_model_ contains_ACC/MATLAB Function5 ==
  settings: updateMethod=DISCRETE  sampleTime=sampleTime
  data: u input; RelDist output
function RelDist = fcn(u)

for i = 1:5
    RelDist = 9999;
end

RelDist = u;

== matlab function Older_model_ contains_ACC/MATLAB Function6 ==
  data: u input; y output Bus: Actors; vehicleID input
function y = fcn(u,vehicleID)

y = u.Actors(vehicleID);

== matlab function Older_model_ contains_ACC/Subsystem6/MATLAB Function ==
  data: modulated input; signal output; SNR input
function signal = PRO_error(modulated, SNR)

signal = awgn(modulated,SNR);

== matlab function Older_model_ contains_ACC/Subsystem6/MATLAB Function1 ==
  data: busActors3Test1 input; Actor output int16 size=15; VehicleID input; VehicleData output Bus: Actors; EgoData input Bus: Actors; counter output; SNR output
  events: trigger input RISING_EDGE_EVENT
function [Actor, VehicleData, counter, SNR]  = convBus2IntVector(busActors3Test1, VehicleID, EgoData)

% Data extracted from actorss bus

%ActorId = BusActors1Actors.Actors(ActorID).ActorID(1:1);
numActors = busActors3Test1.NumActors;
%time = busActors3Test1.Time;
time = busActors3Test1.Time;

ActorID = VehicleID;

posX = busActors3Test1.Actors(ActorID).Position(1:1);
posY = busActors3Test1.Actors(ActorID).Position(2:2);
posZ = busActors3Test1.Actors(ActorID).Position(3:3);
vPos = [posX posY posZ];

vX = busActors3Test1.Actors(ActorID).Velocity(1:1);
vY = busActors3Test1.Actors(ActorID).Velocity(2:2);
vZ = busActors3Test1.Actors(ActorID).Velocity(3:3);

roll = busActors3Test1.Actors(ActorID).Roll(1:1);
pitch = busActors3Test1.Actors(ActorID).Pitch(1:1);
yaw = busActors3Test1.Actors(ActorID).Yaw(1:1);


angularVelocityX = busActors3Test1.Actors(ActorID).AngularVelocity(1:1);
angularVelocityY = busActors3Test1.Actors(ActorID).AngularVelocity(2:2);
angularVelocityZ = busActors3Test1.Actors(ActorID).AngularVelocity(3:3);

VehicleData = busActors3Test1.Actors(ActorID);


%% Converting the data

ActorID = int16(ActorID);

posMultip = 10;
posX = int16(round(posMultip*posX));
posY = int16(round(posMultip*posY));
posZ = int16(round(posMultip*posZ));

velMultip = 50;
vX = int16(round(velMultip * vX));
vY = int16(round(velMultip * vY));
vZ = int16(round(velMultip * vZ));

rpyMultip = 50;
roll = int16(round(rpyMultip * roll));
pitch = int16(round(rpyMultip * pitch));
yaw = int16(round(rpyMultip * yaw));

angvelMultip = 50;
angularVelocityX = int16(round(angvelMultip * angularVelocityX));
angularVelocityY = int16(round(angvelMultip * angularVelocityY));
angularVelocityZ = int16(round(angvelMultip * angularVelocityZ));


% Output vector
%zerosVector = zeros(9,1);

intVector = [numActors; time; ActorID; posX; posY; posZ; vX; vY; vZ; roll; pitch; yaw; angularVelocityX; angularVelocityY; angularVelocityZ];



%% Pathloss (freespace)

EgoPos = EgoData.Position;
dist = norm(vPos - EgoPos);

fc = 5.9*10^9;  % Carrier frequency
lambda = physconst('LightSpeed')/fc;

PL = fspl(dist, lambda);

Pt_dBm = 33;    % [dBm] Transmission power; maximum permissible transmit power level
sigma = rand(1) + 3.2;  % [3.7 +- 0.5] Variance of the shadowing effect in the wireless communication channel
                        % shadowing follows a log-normal random distribution
X = 2*rand(1)-1;       % random variable following a normal distribution with mean 0 and standard deviation 1
SH = sigma * X;

Pr = Pt_dBm - PL - SH;

P_SEN = -60;

%ZeroActors = int16(zeros(15,1));

counter = 0;
% storedPacket = int16(nan(15,1));
% 
% if Pr > P_SEN
%     Actor = intVector;
%     storedPacket = intVector;
%     counter = 0;
% elseif counter < 10
%     Actor = storedPacket;
%     counter = counter + 1;
% else 
%     Actor = int16(nan(15,1));
% end
%disp(storedPacket)


persistent prev_value;
if isempty(prev_value)
    prev_value = int16(nan(15,1)); % Initialize to a default value
end

if Pr > P_SEN
    Actor = intVector;
    prev_value = intVector;
    counter = 0;
elseif counter < 1
    Actor = prev_value;
    counter = counter + 1;
end

%% SNR

F = 6; % [dB] Noise figure
k = physconst('Boltzmann'); % Boltzmann 
T = 300; % [K] Absolut temperature

N0 = F*k*T;

SNR = Pt_dBm - N0;


%% Packet counter
counter = 0;

if (Pr > P_SEN)
    counter = counter + 1;
end


end

== matlab function Older_model_ contains_ACC/Subsystem7/MATLAB Function ==
  data: modulated input; signal output; SNR input
function signal = PRO_error(modulated, SNR)

signal = awgn(modulated,SNR);

== matlab function Older_model_ contains_ACC/Subsystem7/MATLAB Function1 ==
  data: busActors3Test1 input; Actor output int16 size=15; VehicleID input; VehicleData output Bus: Actors; EgoData input Bus: Actors; counter output; SNR output
  events: trigger input RISING_EDGE_EVENT
function [Actor, VehicleData, counter, SNR]  = convBus2IntVector(busActors3Test1, VehicleID, EgoData)

% Data extracted from actorss bus

%ActorId = BusActors1Actors.Actors(ActorID).ActorID(1:1);
numActors = busActors3Test1.NumActors;
%time = busActors3Test1.Time;
time = busActors3Test1.Time;

ActorID = VehicleID;

posX = busActors3Test1.Actors(ActorID).Position(1:1);
posY = busActors3Test1.Actors(ActorID).Position(2:2);
posZ = busActors3Test1.Actors(ActorID).Position(3:3);
vPos = [posX posY posZ];

vX = busActors3Test1.Actors(ActorID).Velocity(1:1);
vY = busActors3Test1.Actors(ActorID).Velocity(2:2);
vZ = busActors3Test1.Actors(ActorID).Velocity(3:3);

roll = busActors3Test1.Actors(ActorID).Roll(1:1);
pitch = busActors3Test1.Actors(ActorID).Pitch(1:1);
yaw = busActors3Test1.Actors(ActorID).Yaw(1:1);


angularVelocityX = busActors3Test1.Actors(ActorID).AngularVelocity(1:1);
angularVelocityY = busActors3Test1.Actors(ActorID).AngularVelocity(2:2);
angularVelocityZ = busActors3Test1.Actors(ActorID).AngularVelocity(3:3);

VehicleData = busActors3Test1.Actors(ActorID);


%% Converting the data

ActorID = int16(ActorID);

posMultip = 10;
posX = int16(round(posMultip*posX));
posY = int16(round(posMultip*posY));
posZ = int16(round(posMultip*posZ));

velMultip = 50;
vX = int16(round(velMultip * vX));
vY = int16(round(velMultip * vY));
vZ = int16(round(velMultip * vZ));

rpyMultip = 50;
roll = int16(round(rpyMultip * roll));
pitch = int16(round(rpyMultip * pitch));
yaw = int16(round(rpyMultip * yaw));

angvelMultip = 50;
angularVelocityX = int16(round(angvelMultip * angularVelocityX));
angularVelocityY = int16(round(angvelMultip * angularVelocityY));
angularVelocityZ = int16(round(angvelMultip * angularVelocityZ));


% Output vector
%zerosVector = zeros(9,1);

intVector = [numActors; time; ActorID; posX; posY; posZ; vX; vY; vZ; roll; pitch; yaw; angularVelocityX; angularVelocityY; angularVelocityZ];



%% Pathloss (freespace)

EgoPos = EgoData.Position;
dist = norm(vPos - EgoPos);

fc = 5.9*10^9;  % Carrier frequency
lambda = physconst('LightSpeed')/fc;

PL = fspl(dist, lambda);

Pt_dBm = 33;    % [dBm] Transmission power; maximum permissible transmit power level
sigma = rand(1) + 3.2;  % [3.7 +- 0.5] Variance of the shadowing effect in the wireless communication channel
                        % shadowing follows a log-normal random distribution
X = 2*rand(1)-1;       % random variable following a normal distribution with mean 0 and standard deviation 1
SH = sigma * X;

Pr = Pt_dBm - PL - SH;

P_SEN = -60;

%ZeroActors = int16(zeros(15,1));

counter = 0;
% storedPacket = int16(nan(15,1));
% 
% if Pr > P_SEN
%     Actor = intVector;
%     storedPacket = intVector;
%     counter = 0;
% elseif counter < 10
%     Actor = storedPacket;
%     counter = counter + 1;
% else 
%     Actor = int16(nan(15,1));
% end
%disp(storedPacket)


persistent prev_value;
if isempty(prev_value)
    prev_value = int16(nan(15,1)); % Initialize to a default value
end

if Pr > P_SEN
    Actor = intVector;
    prev_value = intVector;
    counter = 0;
elseif counter < 1
    Actor = prev_value;
    counter = counter + 1;
end

%% SNR

F = 6; % [dB] Noise figure
k = physconst('Boltzmann'); % Boltzmann 
T = 300; % [K] Absolut temperature

N0 = F*k*T;

SNR = Pt_dBm - N0;


%% Packet counter
counter = 0;

if (Pr > P_SEN)
    counter = counter + 1;
end


end

== matlab function Older_model_ contains_ACC/Subsystem/MATLAB Function1 ==
  settings: sampleTime=inherited
  data: busActors3Test1 input; Actor output int16 size=15; VehicleID input; VehicleData output Bus: Actors; EgoData input Bus: Actors; counter output; SNR output
  events: trigger input RISING_EDGE_EVENT
function [Actor, VehicleData, counter, SNR]  = convBus2IntVector(busActors3Test1, VehicleID, EgoData)

% Data extracted from actorss bus

%ActorId = BusActors1Actors.Actors(ActorID).ActorID(1:1);
numActors = busActors3Test1.NumActors;
%time = busActors3Test1.Time;
time = busActors3Test1.Time;

ActorID = VehicleID;

posX = busActors3Test1.Actors(ActorID).Position(1:1);
posY = busActors3Test1.Actors(ActorID).Position(2:2);
posZ = busActors3Test1.Actors(ActorID).Position(3:3);
vPos = [posX posY posZ];

vX = busActors3Test1.Actors(ActorID).Velocity(1:1);
vY = busActors3Test1.Actors(ActorID).Velocity(2:2);
vZ = busActors3Test1.Actors(ActorID).Velocity(3:3);

roll = busActors3Test1.Actors(ActorID).Roll(1:1);
pitch = busActors3Test1.Actors(ActorID).Pitch(1:1);
yaw = busActors3Test1.Actors(ActorID).Yaw(1:1);


angularVelocityX = busActors3Test1.Actors(ActorID).AngularVelocity(1:1);
angularVelocityY = busActors3Test1.Actors(ActorID).AngularVelocity(2:2);
angularVelocityZ = busActors3Test1.Actors(ActorID).AngularVelocity(3:3);

VehicleData = busActors3Test1.Actors(VehicleID);


%% Converting the data

ActorID = int16(ActorID);

posMultip = 10;
posX = int16(round(posMultip*posX));
posY = int16(round(posMultip*posY));
posZ = int16(round(posMultip*posZ));

velMultip = 50;
vX = int16(round(velMultip * vX));
vY = int16(round(velMultip * vY));
vZ = int16(round(velMultip * vZ));

rpyMultip = 50;
roll = int16(round(rpyMultip * roll));
pitch = int16(round(rpyMultip * pitch));
yaw = int16(round(rpyMultip * yaw));

angvelMultip = 50;
angularVelocityX = int16(round(angvelMultip * angularVelocityX));
angularVelocityY = int16(round(angvelMultip * angularVelocityY));
angularVelocityZ = int16(round(angvelMultip * angularVelocityZ));


% Output vector
%zerosVector = zeros(9,1);

intVector = [numActors; time; ActorID; posX; posY; posZ; vX; vY; vZ; roll; pitch; yaw; angularVelocityX; angularVelocityY; angularVelocityZ];



%% Pathloss (freespace)

EgoPos = EgoData.Position;
dist = norm(vPos - EgoPos);

fc = 5.9e9;  % Carrier frequency
lambda = physconst('LightSpeed')/fc;

PL = fspl(dist, lambda);

Pt_dBm = 33;    % [dBm] Transmission power; maximum permissible transmit power level
sigma = rand(1) + 3.2;  % [3.7 +- 0.5] Variance of the shadowing effect in the wireless communication channel
                        % shadowing follows a log-normal random distribution
X = 2*rand(1)-1;      % random variable following a normal distribution with mean 0 and standard deviation 1
SH = sigma * X;

Pr = Pt_dBm - PL - SH;

P_SEN = -60;

%ZeroActors = int16(zeros(15,1));
% 
counter = 0;
% storedPacket = int16(nan(15,1));
% 
% if Pr > P_SEN
%     Actor = intVector;
%     storedPacket = intVector;
%     counter = 0;
% elseif counter < 10
%     Actor = storedPacket;
%     counter = counter + 1;
% end


%disp(storedPacket)


persistent prev_value;
if isempty(prev_value)
    prev_value = int16(nan(15,1)); % Initialize to a default value
end

if Pr > P_SEN
    Actor = intVector;
    prev_value = intVector;
    counter = 0;
elseif counter < 1
    Actor = prev_value;
    counter = counter + 1;
end

%% SNR

F = 6; % [dB] Noise figure
k = physconst('Boltzmann'); % Boltzmann állandó
T = 300; % [K] Abszolút hőmérséklet

N0 = F*k*T;

SNR = Pt_dBm - N0;


%% Packet counter
counter = 0;

if (Pr > P_SEN)
    counter = counter + 1;
end


end

== matlab function Older_model_ contains_ACC/Subsystem3/MATLAB Function2 ==
  settings: sampleTime=sampleTime
  data: input input; Actors output
function Actors = getRealValues(input) 

modulated = input;

NumActors = modulated(1,:);
Time = modulated(2,:);

ActorID = modulated(3,1);

posMultip = 10;  % 10
posX = (modulated(4,:)/posMultip);
posY = (modulated(5,:)/posMultip);
posZ = (modulated(6,:)/posMultip);

velMultip = 50;  % 50
vX = (modulated(7,:)/velMultip);
vY = (modulated(8,:)/velMultip);
vZ = (modulated(9,:)/velMultip);

rpyMultip = 50;  % 50
Roll = (modulated(10,:)/rpyMultip);
Pitch = (modulated(11,:)/rpyMultip);
Yaw = (modulated(12,:)/rpyMultip);

angvelMultip = 50;  % 50
angularVelocityX = (modulated(13,:)/angvelMultip);
angularVelocityY = (modulated(14,:)/angvelMultip);
angularVelocityZ = (modulated(15,:)/angvelMultip);

% Velocity = [vX vY vZ];
% Position = [posX posY posZ];
% AngularVelocity = [angularVelocityX; angularVelocityY; angularVelocityZ];


%Actors = [NumActors; Time; ActorID; Position; Velocity; Roll; Pitch; Yaw; AngularVelocity];
Actors = [NumActors; Time; ActorID; posX; posY; posZ; vX; vY; vZ; Roll; Pitch; Yaw; angularVelocityX; angularVelocityY; angularVelocityZ];


end

== matlab function Older_model_ contains_ACC/Subsystem3/Subsystem1/MATLAB Function3 ==
  settings: updateMethod=DISCRETE
  data: input input; output output
function output = removeZeros(input)

output = input(1:40,:,:);

end
